simulink model "RC_Schaltung_Reihe"  (R2025b)
settings: Solver=VariableStepAuto  StartTime=0.0  StopTime=10.0  RelTol=1e-3
settings Model: Creator=georg  LastModifiedBy=georg

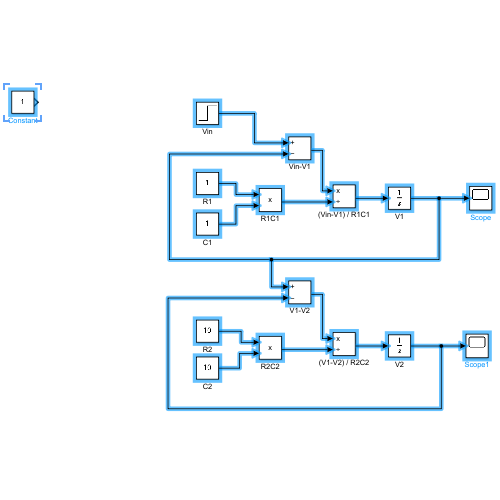
[thumbnail: Simulink's stored preview of the top-level diagram]
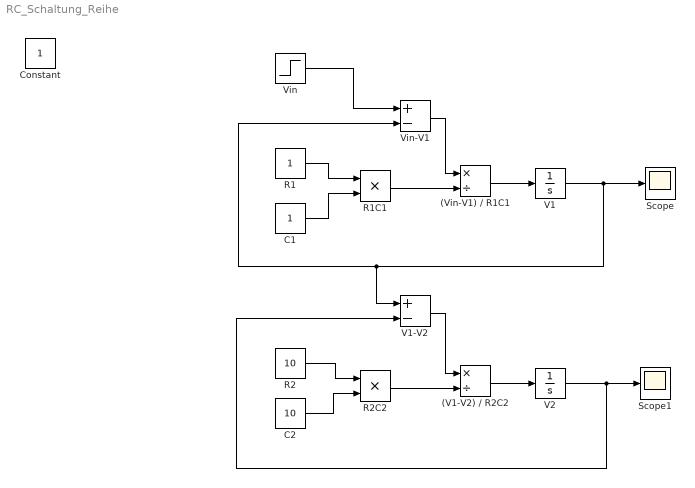
== system RC_Schaltung_Reihe ==
  (V1-V2) / R2C2 : Product  Inputs=*/
  (Vin-V1) / R1C1 : Product  Inputs=*/
  C1 : Constant
  C2 : Constant  Value=10
  Constant : Constant
  R1 : Constant
  R1C1 : Product
  R2 : Constant  Value=10
  R2C2 : Product
  Scope : Scope
  Scope1 : Scope
  V1 : Integrator
  V1-V2 : Sum  Inputs=+-
  V2 : Integrator
  Vin : Step  SampleTime=0
  Vin-V1 : Sum  Inputs=+-
  wires:
  R1/1 -> R1C1/1
  C1/1 -> R1C1/2
  R2/1 -> R2C2/1
  C2/1 -> R2C2/2
  R1C1/1 -> (Vin-V1) / R1C1/2
  R2C2/1 -> (V1-V2) / R2C2/2
  Vin/1 -> Vin-V1/1
  Vin-V1/1 -> (Vin-V1) / R1C1/1
  (Vin-V1) / R1C1/1 -> V1/1
  V1/1 -> V1-V2/1, Vin-V1/2, Scope/1
  (V1-V2) / R2C2/1 -> V2/1
  V2/1 -> Scope1/1, V1-V2/2
  V1-V2/1 -> (V1-V2) / R2C2/1
